simulink model "Simulink"  (R2024b)
settings: Solver=VariableStepAuto  StartTime=0.0  StopTime=10.0  RelTol=1e-3
values from neighbouring files (symbols this model uses):
  A = [0 0 0 0 0 0 0 -35.31 1 0 -9.431 0 ... (16 elements, 4x4)]    [GruaWorkspace.mat]    (also in grua.mat = [0 0 0 0 0 0 0 -35.3130710133 1 0 -9.69067245938 0 ... (16 e)
  B = [0 -0.2969 0.23092 -1.466]    [GruaWorkspace.mat]    (also in grua.mat = [0 -0.296894785399 0.236071876692 -1.46592019656])
  C1 = [1 0 0 0]    [GruaWorkspace.mat]    (also in grua.mat = [1  0  0  0; 0  1  0  0])
  K = [11.5306093495 -2.18400239767 -4.77096681502 -2.1884524864]    [GruaWorkspace.mat]    (also in grua.mat = [11.2779924086 -1.98610202692 -5.28014178733 -2.15028681626])
  Ki = 4.2310165345    [GruaWorkspace.mat]    (also in grua.mat = 4.13832170273)
libraries: simulink x1
settings Model: Creator=wilbe  LastModifiedBy=wilbe
settings SolverCC: ZeroCrossAlgorithm=Adaptive
settings DebuggingCC: IgnoredZcDiagnostic=none

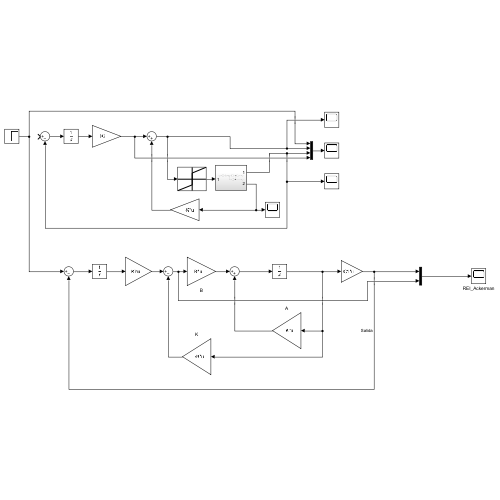
[thumbnail: Simulink's stored preview of the top-level diagram]
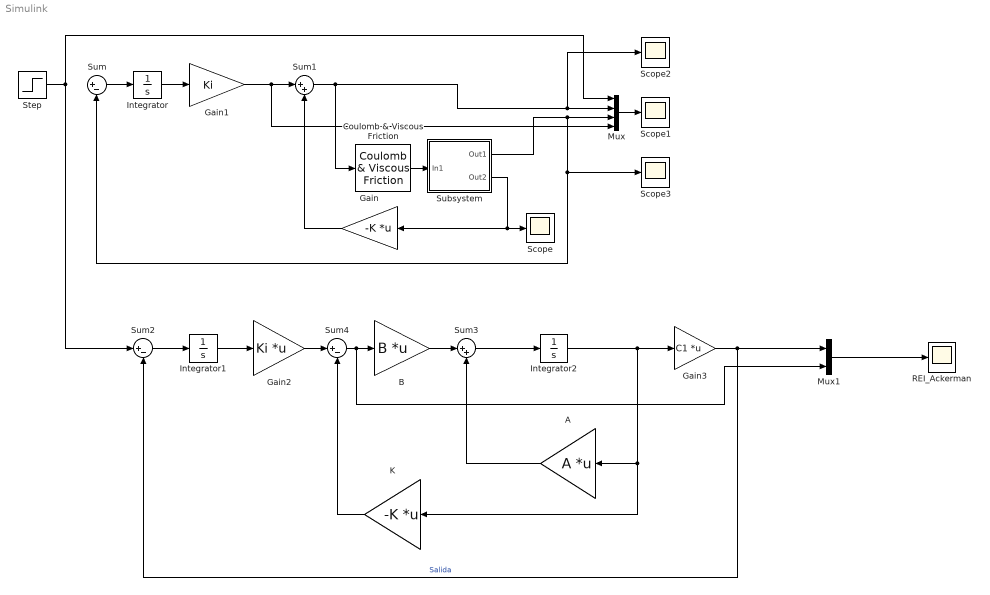
== system Simulink ==
  A : Gain  Gain=A  Multiplication=Matrix(K*u)
  B : Gain  Gain=B  Multiplication=Matrix(K*u)
  Coulomb & Viscous Friction : simulink/Discontinuities/Coulomb & Viscous Friction  offset=[1 3 2 0]  gain=1
  Gain : Gain  Gain=-K  Multiplication=Matrix(K*u)
  Gain1 : Gain  Gain=Ki
  Gain2 : Gain  Gain=Ki  Multiplication=Matrix(K*u)
  Gain3 : Gain  Gain=C1  Multiplication=Matrix(K*u)
  Integrator : Integrator
  Integrator1 : Integrator
  Integrator2 : Integrator
  K : Gain  Gain=-K  Multiplication=Matrix(K*u)
  Mux : Mux
  Mux1 : Mux  Inputs=2
  REI_Ackerman : Scope
  Scope{,1..3} (4 alike) : Scope
  Step : Step  SampleTime=0
  Subsystem : Subsystem
  Sum : Sum  Inputs=|+-
  Sum1 : Sum  Inputs=|++
  Sum2 : Sum  Inputs=|+-
  Sum3 : Sum  Inputs=|++
  Sum4 : Sum  Inputs=|+-
  wires:
  Sum/1 -> Integrator/1
  Integrator/1 -> Gain1/1
  Gain1/1 -> Mux/4, Sum1/1
  Sum1/1 -> Mux/2, Scope2/1, Coulomb & Viscous Friction/1
  Mux/1 -> Scope1/1
  Coulomb & Viscous Friction/1 -> Subsystem/1(In1)
  Subsystem/1(Out1) -> Mux/3, Scope3/1, Sum/2
  Subsystem/2(Out2) -> Gain/1, Scope/1
  Gain/1 -> Sum1/2
  Step/1 -> Sum2/1, Mux/1
  Sum2/1 -> Integrator1/1
  Integrator2/1 -> K/1, A/1, Gain3/1
  Sum3/1 -> Integrator2/1
  Integrator1/1 -> Gain2/1
  Gain2/1 -> Sum4/1
  A/1 -> Sum3/2
  K/1 -> Sum4/2
  Mux1/1 -> REI_Ackerman/1
  Gain3/1 -> Mux1/1, Sum2/2  "Salida"
  Sum4/1 -> Mux1/2, B/1
  B/1 -> Sum3/1

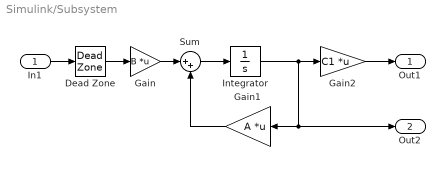
== system Simulink/Subsystem ==
  In1 : Inport
  Dead Zone : DeadZone  UpperValue=0.6
  Gain : Gain  Gain=B  Multiplication=Matrix(K*u)
  Gain1 : Gain  Gain=A  Multiplication=Matrix(K*u)
  Gain2 : Gain  Gain=C1  Multiplication=Matrix(K*u)
  Integrator : Integrator
  Sum : Sum  Inputs=|++
  Out1 : Outport
  Out2 : Outport  Port=2
  wires:
  In1/1 -> Dead Zone/1
  Dead Zone/1 -> Gain/1
  Gain/1 -> Sum/1
  Gain1/1 -> Sum/2
  Sum/1 -> Integrator/1
  Integrator/1 -> Gain2/1, Out2/1, Gain1/1
  Gain2/1 -> Out1/1
